simulink model "extctrl_example20200707"  (Simulink 7.9)
settings: Solver=FixedStepDiscrete  StartTime=0.0  StopTime=10.0  RelTol=1e-3
undefined symbols (not defined in the file): amplitude, frequency, h
libraries: simulink_extras x1
settings Model: Creator=jjwang  LastModifiedBy=julian  ExtModeAutoUpdateStatusClock=off  TunableVars=amplitude,frequency  TunableVarsStorageClass=Auto,Auto  TunableVarsTypeQualifier=,
settings DataIOCC: SaveOutput=off  SaveTime=off  SignalLoggingName=sigsOut
settings OptimizationCC: BooleanDataType=off  InlineParams=on  RollThreshold=8  InitFltsAndDblsToZero=on
settings DebuggingCC: SaveWithParameterizedLinksMsg=none  SignalResolutionControl=TryResolveAllWithWarning  SolverPrmCheckMsg=none  MultiTaskDSMMsg=warning  MultiTaskCondExecSysMsg=none  FcnCallInpInsideContextMsg=Use local settings  StrictBusMsg=None
settings HardwareCC: ProdHWDeviceType=Specified  TargetHWDeviceType=32-bit Generic  ProdEqTarget=off
settings RTWCC: SystemTargetFile=rtw2orca.tlc  TemplateMakefile=rtw2orca.tmf  Description=RTW2ORCA Real-Time Target  RetainRTWFile=on  ProcessScript=rtw2orca_make_rtw_hook
settings CodeAppCC: ForceParamTrailComments=on  MaxIdLength=128
settings STFCustomTargetCC: TargetFcnLib=ansi_tfl_tmw.mat  CodeReplacementLibrary=ANSI_C  ModelReferenceCompliant=off  GeneratePreprocessorConditionals=Disable all  MatFileLogging=on  SystemTargetFile=rtw2orca.tlc
settings CustomProperty: DataType=string  Value=ext2irb irb2ext

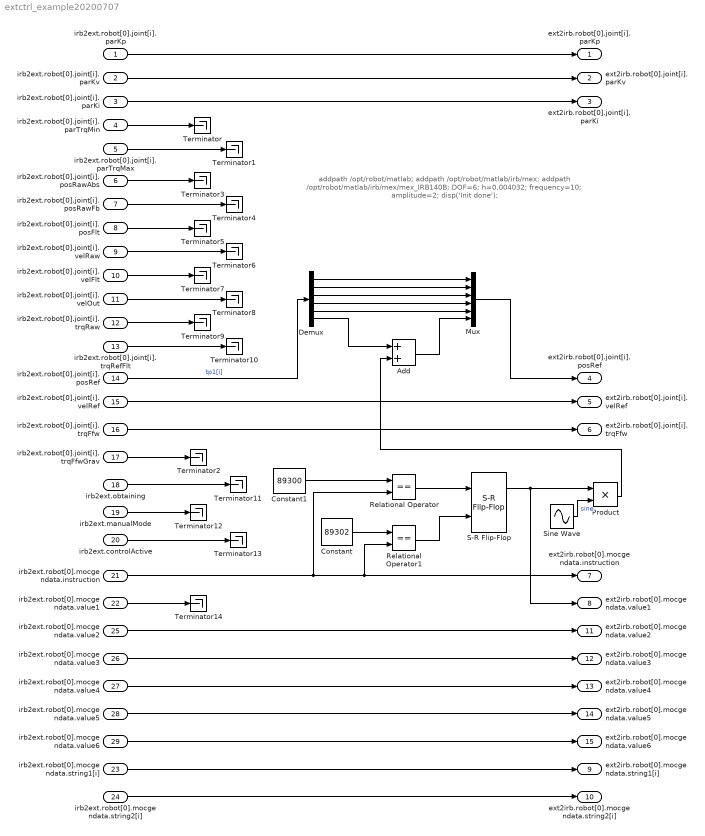
== system extctrl_example20200707 ==
  note: addpath /opt/robot/matlab;
      | addpath /opt/robot/matlab/irb/mex;
      | addpath /opt/robot/matlab/irb/mex/mex_IRB140B;
      |
      | DOF=6;
      | h=0.004032;
      | frequency=10;
      | amplitude=2;
      | disp('Init done');
  irb2ext.robot[0].joint[i].parKp : Inport  OutDataTypeStr=double  PortDimensions=DOF
  irb2ext.robot[0].joint[i].parKv : Inport  Port=2  OutDataTypeStr=double  PortDimensions=DOF
  irb2ext.robot[0].joint[i].parKi : Inport  Port=3  PortDimensions=DOF
  irb2ext.robot[0].joint[i].parTrqMin : Inport  Port=4  PortDimensions=DOF
  irb2ext.robot[0].joint[i].parTrqMax : Inport  Port=5  PortDimensions=DOF
  irb2ext.robot[0].joint[i].posRawAbs : Inport  Port=6  PortDimensions=DOF
  irb2ext.robot[0].joint[i].posRawFb : Inport  Port=7  PortDimensions=DOF
  irb2ext.robot[0].joint[i].posFlt : Inport  Port=8  PortDimensions=DOF
  irb2ext.robot[0].joint[i].velRaw : Inport  Port=9  PortDimensions=DOF
  irb2ext.robot[0].joint[i].velFlt : Inport  Port=10  PortDimensions=DOF
  irb2ext.robot[0].joint[i].velOut : Inport  Port=11  PortDimensions=DOF
  irb2ext.robot[0].joint[i].trqRaw : Inport  Port=12  PortDimensions=DOF
  irb2ext.robot[0].joint[i].trqRefFlt : Inport  Port=13  PortDimensions=DOF
  irb2ext.robot[0].joint[i].posRef : Inport  Port=14  PortDimensions=DOF
  irb2ext.robot[0].joint[i].velRef : Inport  Port=15  PortDimensions=DOF
  irb2ext.robot[0].joint[i].trqFfw : Inport  Port=16  PortDimensions=DOF
  irb2ext.robot[0].joint[i].trqFfwGrav : Inport  Port=17  PortDimensions=DOF
  irb2ext.obtaining : Inport  Port=18  PortDimensions=1
  irb2ext.manualMode : Inport  Port=19  PortDimensions=1
  irb2ext.controlActive : Inport  Port=20  PortDimensions=1
  irb2ext.robot[0].mocgendata.instruction : Inport  Port=21  PortDimensions=1
  irb2ext.robot[0].mocgendata.value1 : Inport  Port=22  PortDimensions=1
  irb2ext.robot[0].mocgendata.string1[i] : Inport  Port=23  PortDimensions=20
  irb2ext.robot[0].mocgendata.string2[i] : Inport  Port=24  PortDimensions=20
  irb2ext.robot[0].mocgendata.value2 : Inport  Port=25  PortDimensions=1
  irb2ext.robot[0].mocgendata.value3 : Inport  Port=26  PortDimensions=1
  irb2ext.robot[0].mocgendata.value4 : Inport  Port=27  PortDimensions=1
  irb2ext.robot[0].mocgendata.value5 : Inport  Port=28  PortDimensions=1
  irb2ext.robot[0].mocgendata.value6 : Inport  Port=29  PortDimensions=1
  Add : Sum
  Constant : Constant  Value=89302
  Constant1 : Constant  Value=89300
  Demux : Demux  Outputs=6
  Mux : Mux  Inputs=6
  Product : Product  RndMeth=Zero
  Relational Operator : RelationalOperator  Operator===  OutDataTypeStr=boolean
  Relational Operator1 : RelationalOperator  Operator===  OutDataTypeStr=boolean
  S-R Flip-Flop : simulink_extras/Flip Flops/S-R Flip-Flop  initial_condition=1
  Sine Wave : Sin  Amplitude=amplitude  Frequency=frequency  Samples=frequency  SampleTime=h
  Terminator{,1..14} (15 alike) : Terminator
  ext2irb.robot[0].joint[i].parKp : Outport  PortDimensions=DOF
  ext2irb.robot[0].joint[i].parKv : Outport  Port=2  PortDimensions=DOF
  ext2irb.robot[0].joint[i].parKi : Outport  Port=3  PortDimensions=DOF
  ext2irb.robot[0].joint[i].posRef : Outport  Port=4  PortDimensions=DOF
  ext2irb.robot[0].joint[i].velRef : Outport  Port=5  PortDimensions=DOF
  ext2irb.robot[0].joint[i].trqFfw : Outport  Port=6  PortDimensions=DOF
  ext2irb.robot[0].mocgendata.instruction : Outport  Port=7  PortDimensions=1
  ext2irb.robot[0].mocgendata.value1 : Outport  Port=8  PortDimensions=1
  ext2irb.robot[0].mocgendata.string1[i] : Outport  Port=9  PortDimensions=20
  ext2irb.robot[0].mocgendata.string2[i] : Outport  Port=10  PortDimensions=20
  ext2irb.robot[0].mocgendata.value2 : Outport  Port=11  PortDimensions=1
  ext2irb.robot[0].mocgendata.value3 : Outport  Port=12  PortDimensions=1
  ext2irb.robot[0].mocgendata.value4 : Outport  Port=13  PortDimensions=1
  ext2irb.robot[0].mocgendata.value5 : Outport  Port=14  PortDimensions=1
  ext2irb.robot[0].mocgendata.value6 : Outport  Port=15  PortDimensions=1
  wires:
  irb2ext.robot[0].joint[i].parKv/1 -> ext2irb.robot[0].joint[i].parKv/1
  irb2ext.robot[0].joint[i].parKp/1 -> ext2irb.robot[0].joint[i].parKp/1
  irb2ext.robot[0].joint[i].parKi/1 -> ext2irb.robot[0].joint[i].parKi/1
  irb2ext.robot[0].joint[i].parTrqMin/1 -> Terminator/1
  irb2ext.robot[0].joint[i].parTrqMax/1 -> Terminator1/1
  irb2ext.robot[0].joint[i].velRef/1 -> ext2irb.robot[0].joint[i].velRef/1
  irb2ext.robot[0].joint[i].trqFfw/1 -> ext2irb.robot[0].joint[i].trqFfw/1
  irb2ext.robot[0].joint[i].trqFfwGrav/1 -> Terminator2/1
  irb2ext.robot[0].joint[i].posRawAbs/1 -> Terminator3/1
  irb2ext.robot[0].joint[i].posRawFb/1 -> Terminator4/1
  irb2ext.robot[0].joint[i].posFlt/1 -> Terminator5/1
  irb2ext.robot[0].joint[i].velRaw/1 -> Terminator6/1
  irb2ext.robot[0].joint[i].velFlt/1 -> Terminator7/1
  irb2ext.robot[0].joint[i].velOut/1 -> Terminator8/1
  irb2ext.robot[0].joint[i].trqRaw/1 -> Terminator9/1
  irb2ext.robot[0].joint[i].trqRefFlt/1 -> Terminator10/1
  irb2ext.robot[0].joint[i].posRef/1 -> Demux/1  "tp1[i]"
  Mux/1 -> ext2irb.robot[0].joint[i].posRef/1
  Demux/1 -> Mux/1
  Demux/2 -> Mux/2
  Demux/3 -> Mux/3
  Demux/4 -> Mux/4
  Demux/5 -> Mux/5
  Demux/6 -> Add/1
  Add/1 -> Mux/6
  irb2ext.obtaining/1 -> Terminator11/1
  irb2ext.manualMode/1 -> Terminator12/1
  irb2ext.controlActive/1 -> Terminator13/1
  irb2ext.robot[0].mocgendata.instruction/1 -> Relational Operator/2, ext2irb.robot[0].mocgendata.instruction/1, Relational Operator1/2
  irb2ext.robot[0].mocgendata.string1[i]/1 -> ext2irb.robot[0].mocgendata.string1[i]/1
  irb2ext.robot[0].mocgendata.string2[i]/1 -> ext2irb.robot[0].mocgendata.string2[i]/1
  irb2ext.robot[0].mocgendata.value2/1 -> ext2irb.robot[0].mocgendata.value2/1
  irb2ext.robot[0].mocgendata.value3/1 -> ext2irb.robot[0].mocgendata.value3/1
  irb2ext.robot[0].mocgendata.value4/1 -> ext2irb.robot[0].mocgendata.value4/1
  irb2ext.robot[0].mocgendata.value5/1 -> ext2irb.robot[0].mocgendata.value5/1
  irb2ext.robot[0].mocgendata.value6/1 -> ext2irb.robot[0].mocgendata.value6/1
  irb2ext.robot[0].mocgendata.value1/1 -> Terminator14/1
  Constant1/1 -> Relational Operator/1
  Constant/1 -> Relational Operator1/1
  Relational Operator/1 -> S-R Flip-Flop/1
  Relational Operator1/1 -> S-R Flip-Flop/2
  S-R Flip-Flop/1 -> ext2irb.robot[0].mocgendata.value1/1, Product/1
  Sine Wave/1 -> Product/2  "sine"
  Product/1 -> Add/2
